simulink model "ControlTest"  (Simulink 7.5)
settings: Solver=ode45  StartTime=0.0  StopTime=0.8  FixedStep=0.001  RelTol=1e-3
undefined symbols (not defined in the file or in its folder): c, g, Ih, Kd, Ki, Kp, mh, rh, Rsma, Xh
libraries: simulink x3
settings Model: Creator=jdcolorado  LastModifiedBy=Administrador
settings SolverCC: ZeroCrossControl=DisableAll
settings OptimizationCC: InitFltsAndDblsToZero=on
settings DebuggingCC: StrictBusMsg=Warning

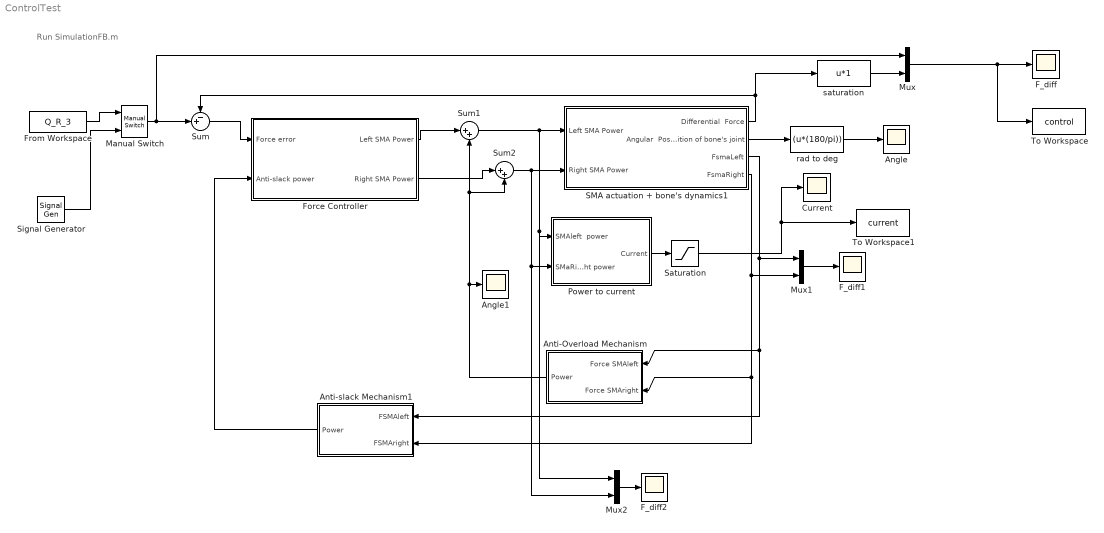
== system ControlTest ==
  note: Run SimulationFB.m
  " Force Controller" : Subsystem
  Angle : Scope
      settings: TimeRange=0.16  YMin=0.351136316872428  YMax=0.374136316872428
  Angle1 : Scope
      settings: YMin=0.3175  YMax=0.375  SaveName=ScopeData5
  Anti-Overload Mechanism : Subsystem
  Anti-slack Mechanism1 : Subsystem
  Current : Scope
      settings: TimeRange=0.35  YMin=0  YMax=0.8
  F_diff : Scope
      settings: TimeRange=0.4  YMin=15  YMax=90  SaveName=ScopeData2
  F_diff1 : Scope
      settings: TimeRange=0.35  YMin=-0.275  YMax=0.275  SaveName=ScopeData3
  F_diff2 : Scope
      settings: YMin=-0.375  YMax=0.175  SaveName=ScopeData4
  From Workspace : FromWorkspace  VariableName=Q_R_3  SampleTime=step  OutputAfterFinalValue=Setting to zero
  Manual Switch : simulink/Signal Routing/Manual Switch  SystemSampleTime=-1  sw=1  action=0  varsize=off
  Mux : Mux  Inputs=2
  Mux1 : Mux  Inputs=2
  Mux2 : Mux  Inputs=2
  Power to current : Subsystem
  SMA actuation + bone's dynamics1 : Subsystem
  Saturation : Saturate  UpperLimit=0.55  LowerLimit=0.04
  Signal Generator : SignalGenerator  WaveForm=square  Amplitude=0.02  Frequency=2
  Sum : Sum  Inputs=-+|
  Sum1 : Sum  Inputs=|++
  Sum2 : Sum  Inputs=|++
  To Workspace : ToWorkspace  VariableName=control  SampleTime=-1  SaveFormat=Structure
  To Workspace1 : ToWorkspace  VariableName=current  SampleTime=-1  SaveFormat=Structure
  rad to deg : MATLABFcn  MATLABFcn=(u*(180/pi))
  saturation : MATLABFcn  MATLABFcn=u*1
  wires:
  Sum/1 -> " Force Controller"/1(Force error)
  SMA actuation + bone's dynamics1/1(Differential  Force) -> Sum/1, saturation/1
  SMA actuation + bone's dynamics1/2(Angular  Position of bone's joint) -> rad to deg/1
  SMA actuation + bone's dynamics1/3(FsmaLeft) -> Mux1/1, Anti-Overload Mechanism/1(Force SMAleft), Anti-slack Mechanism1/1(FSMAleft)
  SMA actuation + bone's dynamics1/4(FsmaRight) -> Mux1/2, Anti-Overload Mechanism/2(Force SMAright), Anti-slack Mechanism1/2(FSMAright)
  " Force Controller"/1(Left SMA Power) -> Sum1/1
  " Force Controller"/2(Right SMA Power) -> Sum2/1
  Anti-slack Mechanism1/1(Power) -> " Force Controller"/2(Anti-slack power)
  rad to deg/1 -> Angle/1
  Mux/1 -> F_diff/1, To Workspace/1
  Manual Switch/1 -> Sum/2, Mux/1
  From Workspace/1 -> Manual Switch/1
  Signal Generator/1 -> Manual Switch/2
  Mux1/1 -> F_diff1/1
  Mux2/1 -> F_diff2/1
  Sum2/1 -> SMA actuation + bone's dynamics1/2(Right SMA Power), Power to current/2(SMaRight power), Mux2/2
  Sum1/1 -> SMA actuation + bone's dynamics1/1(Left SMA Power), Power to current/1(SMAleft  power), Mux2/1
  Anti-Overload Mechanism/1(Power) -> Sum1/2, Sum2/2, Angle1/1
  Power to current/1(Current) -> Saturation/1
  Saturation/1 -> Current/1, To Workspace1/1
  saturation/1 -> Mux/2

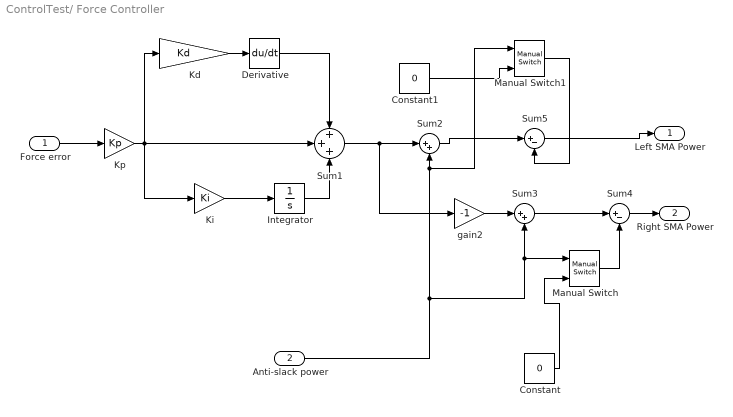
== system ControlTest/ Force Controller ==
  Force error : Inport
  Anti-slack power : Inport  Port=2
  Constant : Constant  Value=0
  Constant1 : Constant  Value=0
  Derivative : Derivative
  Integrator : Integrator
  Kd : Gain  Gain=Kd
  Ki : Gain  Gain=Ki
  Kp : Gain  Gain=Kp
  Manual Switch : simulink/Signal Routing/Manual Switch  SystemSampleTime=-1  sw=1  action=0  varsize=off
  Manual Switch1 : simulink/Signal Routing/Manual Switch  SystemSampleTime=-1  sw=1  action=0  varsize=off
  Sum1 : Sum  Inputs=+++
  Sum2 : Sum  Inputs=|++
  Sum3 : Sum  Inputs=|++
  Sum4 : Sum  Inputs=|+-
  Sum5 : Sum  Inputs=|+-
  gain2 : Gain  Gain=-1
  Left SMA Power : Outport
  Right SMA Power : Outport  Port=2
  wires:
  Force error/1 -> Kp/1
  Kd/1 -> Derivative/1
  Derivative/1 -> Sum1/1
  Kp/1 -> Kd/1, Sum1/2, Ki/1
  Ki/1 -> Integrator/1
  Integrator/1 -> Sum1/3
  Anti-slack power/1 -> Sum3/2, Manual Switch/1, Sum2/2, Manual Switch1/1
  Sum1/1 -> Sum2/1, gain2/1
  gain2/1 -> Sum3/1
  Sum3/1 -> Sum4/1
  Sum4/1 -> Right SMA Power/1
  Sum2/1 -> Sum5/1
  Manual Switch/1 -> Sum4/2
  Sum5/1 -> Left SMA Power/1
  Manual Switch1/1 -> Sum5/2
  Constant/1 -> Manual Switch/2
  Constant1/1 -> Manual Switch1/2

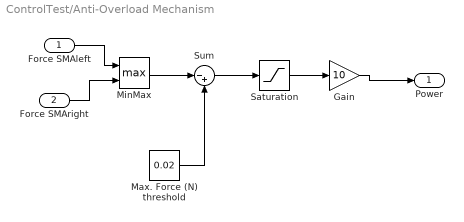
== system ControlTest/Anti-Overload Mechanism ==
  Force SMAleft : Inport
  Force SMAright : Inport  Port=2
  Gain : Gain  Gain=10
  Max. Force (N) threshold : Constant  Value=0.02
  MinMax : MinMax  Function=max  Inputs=2
  Saturation : Saturate  UpperLimit=0
  Sum : Sum  Inputs=|-+
  Power : Outport
  wires:
  Force SMAleft/1 -> MinMax/1
  Force SMAright/1 -> MinMax/2
  MinMax/1 -> Sum/1
  Max. Force (N) threshold/1 -> Sum/2
  Sum/1 -> Saturation/1
  Saturation/1 -> Gain/1
  Gain/1 -> Power/1

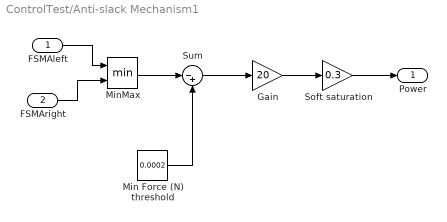
== system ControlTest/Anti-slack Mechanism1 ==
  FSMAleft : Inport
  FSMAright : Inport  Port=2
  Gain : Gain  Gain=20
  Min Force (N) threshold : Constant  Value=0.0002
  MinMax : MinMax  Inputs=2
  Soft saturation : Gain  Gain=0.3
  Sum : Sum  Inputs=|-+
  Power : Outport
  wires:
  FSMAleft/1 -> MinMax/1
  FSMAright/1 -> MinMax/2
  MinMax/1 -> Sum/1
  Min Force (N) threshold/1 -> Sum/2
  Gain/1 -> Soft saturation/1
  Sum/1 -> Gain/1
  Soft saturation/1 -> Power/1

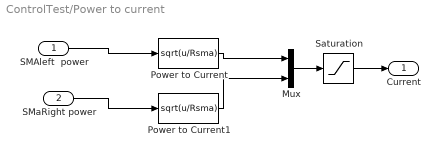
== system ControlTest/Power to current ==
  SMAleft  power : Inport
  SMaRight power : Inport  Port=2
  " Power to Current" : MATLABFcn  MATLABFcn=sqrt(u/Rsma)
  " Power to Current1" : MATLABFcn  MATLABFcn=sqrt(u/Rsma)
  Mux : Mux  Inputs=2
  Saturation : Saturate  UpperLimit=0.8  LowerLimit=0
  Current : Outport
  wires:
  Mux/1 -> Saturation/1
  " Power to Current"/1 -> Mux/1
  " Power to Current1"/1 -> Mux/2
  SMAleft  power/1 -> " Power to Current"/1
  SMaRight power/1 -> " Power to Current1"/1
  Saturation/1 -> Current/1

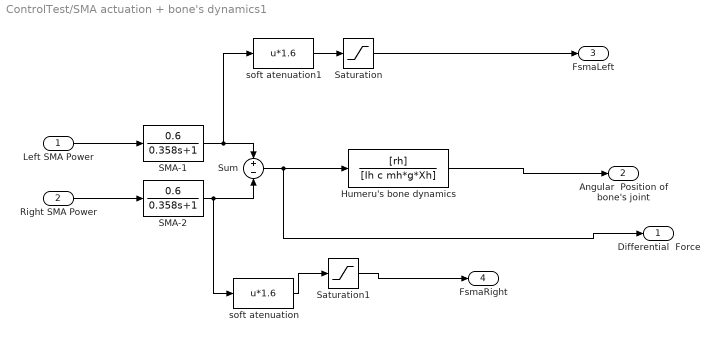
== system ControlTest/SMA actuation + bone's dynamics1 ==
  Left SMA Power : Inport
  Right SMA Power : Inport  Port=2
  Humeru's bone dynamics : TransferFcn  Numerator=[rh]  Denominator=[Ih c mh*g*Xh]
  SMA-1 : TransferFcn  Numerator=[0.6]  Denominator=[0.358 1]
  SMA-2 : TransferFcn  Numerator=[0.6]  Denominator=[0.358 1]
  Saturation : Saturate  UpperLimit=3.5  LowerLimit=-2
  Saturation1 : Saturate  UpperLimit=3.5  LowerLimit=-2
  Sum : Sum  Inputs=+-
  soft atenuation : MATLABFcn  MATLABFcn=u*1.6
  soft atenuation1 : MATLABFcn  MATLABFcn=u*1.6
  Differential  Force : Outport
  Angular  Position of bone's joint : Outport  Port=2
  FsmaLeft : Outport  Port=3
  FsmaRight : Outport  Port=4
  wires:
  Sum/1 -> Humeru's bone dynamics/1, Differential  Force/1
  SMA-2/1 -> Sum/2, soft atenuation/1
  SMA-1/1 -> Sum/1, soft atenuation1/1
  Right SMA Power/1 -> SMA-2/1
  Left SMA Power/1 -> SMA-1/1
  Humeru's bone dynamics/1 -> Angular  Position of bone's joint/1
  Saturation1/1 -> FsmaRight/1
  soft atenuation1/1 -> Saturation/1
  soft atenuation/1 -> Saturation1/1
  Saturation/1 -> FsmaLeft/1
